simulink model "Drone2_simulink_old"  (R2024b)
settings: Solver=ode1be  StartTime=0.0  StopTime=1200  FixedStep=0.001  MaxStep=0.001  MinStep=0.00095  RelTol=1e-3
undefined symbols (not defined in the file): DiscIntNeverNeededParam, Environment, Newton, Raphson, Sim3dSensor, Vehicle, X, Y, Z
libraries: sm_lib x2953, nesl_utility x76, slpidlib x25, simulink x4, eeGeneralControl x4, matrix_library x3, rllib x2, sim3dlib x2, uavsim3dlib x2, dspstat3 x1, SignalEditorBlockLib x1, sharedutil x1
(part 21 of 21)

== matlab function Drone2_simulink_old/Controller (STA-Based)/New Control scheme with STA ==
  settings: updateMethod=DISCRETE  sampleTime=0.001
  data: state input; uc output; desired input; dt parameter; initialz input; tt input; b_out output; e output; ud_new output; parameter parameter; zd output; Env parameter; physical parameter; ld output; vd output; vd_dot output; eta1 output; e_dot output; term output; vzout output; S output; uc1 output; uc2 output; Aout output; AAout output
function [uc,b_out,e,ud_new,zd,ld,vd,vd_dot,eta1,e_dot,term,vzout,S,uc1,uc2,Aout,AAout] = Adaptive_Robust_Controller(state,desired, dt, initialz, tt,parameter,Env, physical)
%%%% defination
% x = states [z,p,u,w,q,lf,lr,lf_dot,lr_dot]
%  m = fixed mass
% m1 = moving mass 
% IB = Inertia tensor of 3*3
% rho = water density
% g = gravity (value in m/s^2)
% AS = syringe area
% ZS = CG location of z axis in each syringe [z1 z2 z3]
% l = length of vehicle/drone
% V = volume of drone
% rb = location of center of buoyancy from body frame [rbx rby rbz];
% RG = inital location of CG from body frame[ rgx rgy rgz];
% desired = target depth and pitch angle and velocities [z z_dot pitch
% pitch_rate]
% MATfile = file of disturnace jonswap.mat
% Parameters:    1x1 structure
%             
% 
% 
% fixed mass
% warning('on','MATLAB:singularMatrix');
% warning('on','MATLAB:nearlySingularMatrix');
% warning('on','MATLAB:illConditionedMatrix');
% dbstop if warning MATLAB:singularMatrix
% dbstop if warning MATLAB:nearlySingularMatrix
% dbstop if warning MATLAB:illConditionedMatrix


persistent isavail b vz vf_trim vb_trim AA A zr_prev


if isempty(isavail)
    b = zeros(2,1);%[0;0];
    A = zeros(2,1);%[0;0];
    AA = zeros(2,1);%[0;0];

    vz = zeros(2,1);%[0;0];
    vf_trim = 0;
    vb_trim = 0;
    zr_prev = desired(1);

    isavail = true;
end





m = physical.m;
IB = physical.IB;
Rsyringe = physical.Rsyringe;
RG = physical.RG;
rb = physical.rb;
l = physical.l;
ZS = physical.ZS;
Sden = physical.Sden;
maxb = physical.maxb;
minb = physical.minb;
rho = Env.rho;
g = abs(Env.g);
MaxBuoyancyVol = physical.MaxBuoyancyVol;
TT = physical.TimeConstant;


Srho = Sden*rho;





%% control gain constants

%<------- Backstepping with disturbance compensator error constant -------->

K1 = parameter.Backcomp.K1;
K2 = parameter.Backcomp.K2;
K22 = parameter.Backcomp.K22;
K2Z = parameter.Backcomp.K2Z;
K1SF = parameter.Backcomp.K1SF;
K2SF = parameter.Backcomp.K2SF;
K3SF =parameter.Backcomp.K3SF;
lb = parameter.Backcomp.lb;
alpha0 = parameter.Backcomp.alpha;
alpha1 = parameter.Backcomp.alpha1;
satphi = parameter.Backcomp.phisat;
satphi1 = parameter.Backcomp.phisat1;
K_trim = parameter.Backcomp.K_Trim;
K_rate = parameter.Backcomp.K_Rate;
EZDB = parameter.Backcomp.EZDB;
KP_trim = parameter.Backcomp.KP_Trim;
KP_rate = parameter.Backcomp.KP_Rate;
ETDB = parameter.Backcomp.ETDB;

%% extra
AS = pi*Rsyringe^2;
arc = [3 5];%[1 3 5];
jr = [3 5];
%% state Identification
% [m11,n1] = size(Dtrue);
% [m22,n22] = size(Ttrue);

Z = state(1);
r=0;y =0;
p = state(2);

u = state(3);
w = state(4);
q = state(5);
vel = [0;0;w];
omega = [0;q;0];



lf = state(6);
lr = state(7);

lf_dot = state(8);
lr_dot = state(9);



vel1 = [w;q];


%% Mass Matrix and coriollis matrix
Mdead = [m*eye(3) -m*skmatrix(RG); m*skmatrix(RG) IB ];  %% dead weight mass mo
Mdead11 = m*eye(3); Mdead12 = -m*skmatrix(RG); Mdead21=-Mdead12; Mdead22 = IB;
Cdead = [zeros(3)  -skmatrix(Mdead11*vel+Mdead12*omega);-skmatrix(Mdead11*vel+Mdead12*omega) -skmatrix(Mdead21*vel+Mdead22*omega)];

[MF1, MF1_dot ,CF1] = M_Mdot_C_Matrix(Srho,Rsyringe,lf,lf_dot,[(l-lf)/2; 0 ; ZS(1)],[-lf_dot/2 ;0 ;0],pi,omega,vel);
[MF2, MF2_dot ,CF2] = M_Mdot_C_Matrix(Srho,Rsyringe,lf,lf_dot,[(l-lf)/2; 0 ; ZS(2)],[-lf_dot/2 ;0 ;0],pi,omega,vel);
[MR, MR_dot ,CR] = M_Mdot_C_Matrix(Srho,Rsyringe,lr,lr_dot,[-(l-lr)/2; 0 ; ZS(3)],[lr_dot/2 ;0 ;0],0,omega,vel);





M = Mdead ;%+ MF1 +MF2 +MR;
C = Cdead;% + CF1 +CF2+ CR;

M_dot = MF1_dot+MF2_dot+MR_dot;


invM =  Mdead\eye(6); %(M+0.001*eye(6))\eye(6);

M = M(arc,arc);
M_dot = M_dot(arc,arc);
invM = invM(arc,arc);
C = C(arc,arc);



%% Making Transformation matrix

Rbw = [cos(p)*cos(y) sin(r)*sin(p)*cos(y)-cos(r)*sin(y)  cos(r)*sin(p)*cos(y)+sin(r)*sin(y);
    cos(p)*sin(y) sin(r)*sin(p)*sin(y)+cos(r)*cos(y)  cos(r)*sin(p)*sin(y)-sin(r)*cos(y);
    -sin(p) sin(r)*cos(p) cos(r)*cos(p)];

% Tbw = [1 sin(r)*tan(p) cos(r)*tan(p); 0 cos(r) -sin(r); 0 sin(r)/cos(p) cos(r)/cos(p)];

% J = [Rbw zeros(3); zeros(3) Tbw]; % 6*6 matrix

% J = J(jr,arc); %2*3 matrix [-sin(p) cos(p) 0; 0 0 1]
% invJ = pinv(J); % or simply j' as J*ji  = I2;      3*2 matrix 

% Jdot = [-cos(p)*q -sin(p)*q 0; 0 0 0];

%% Gravity Matrix
Fgn = [0;0;-Mdead(1,1)*g];
Fbn = [0;0;rho*MaxBuoyancyVol*g];

Fgb = Rbw'*Fgn;
Fbb = Rbw'*Fbn;
% G = -[Fgn+Fbn; cross(RG,Fgn)+cross(rb,Fbn)];
G = -[Fgb+Fbb; cross(RG,Fgb)+cross(rb,Fbb)]; % 6*1 matrix
G = G(arc); % 3*1 vector



%% desired 
if tt<=600
    z = desired(1);
else
    z = -2.5;
end

pd = desired(2);
tau = 4;

%% forward euler case
% zr_dot = (z-zr_prev)/tau;
% zd = zr_prev + dt*zr_dot;
% zr_prev = zd;

%% backward euler case
zd = (zr_prev+(z*dt/tau))/(1+(dt/tau));
zr_dot = (z-zd)/tau;
zr_prev = zd;

%% other desired velocities
eta_dot_d = [zr_dot;desired(4)];
% eta_dot_d = [desired(3);desired(4)];
eta_ddot_d = [desired(5);desired(6)];



        %% Backsteping Algorithm with distubance compensator gain
        e = [Z;p]-[zd;pd];
        
        %% first virtual controller \vd
                
        vd = eta_dot_d -K1*e;

        eta1 = vel1 - vd;
        
        
        e_dot = eta1-K1*e;
        
        vd_dot = eta_ddot_d-K1*e_dot;
        
        
        
        %% second virtual controller u

        % ud_new = (C*vel1+G + Damping - je-K2*eta1+M*vd_dot);
        term = abs(eta1).^0.5.*satfun(eta1,satphi1);



        ud_new = (C*vel1+G-M*(vd_dot-K2*eta1-K22*term+vz));
        % ud_new(1) = clipfunc(ud_new(1),10,0);
        % ud_new(2) = clipfunc(ud_new(2),1.5,-1.5);
        ud_new = reshape(ud_new,2,1);

        vzdot = -K2Z*satfun(eta1,satphi1);

        % vzdot = reshape(vzdot,2,1);
        vz = vz+vzdot*dt;
        vzout = vz;

%% New rule for finding lf and lr
        % K_Trim = 0.002; K_rate = 0.05;
        % EZDB = 0.05;
        % KP_trim = 0.0002; Kp_rate = 0.05;
        % ETDB = 0.05;

        dsum = ud_new(1)/(rho*AS*g);
        vf_fast = 0.25*dsum;
        vb_fast = 0.5*dsum;

        msum = ud_new(2)/(rho*AS*g);
        vf_pitch_fast = 0.25*msum;
        vb_pitch_fast = -0.15*msum; % change 0.5

        adapt_gate = 1/(1+K_rate*abs(eta1(1)));
        if abs(e(1))<EZDB
            adapt_gate = 0.25*adapt_gate;
        end
        dsum_trim = K_trim*e(1)*adapt_gate;

        pitch_gate = 1/(1+KP_rate*abs(eta1(2)));

        if abs(e(2))<ETDB
            pitch_gate = 0.2*pitch_gate;
        end
        msum_trim = KP_trim*e(2)*pitch_gate;

        msum_trim = clipfunc(msum_trim,0.01,-0.01);

        vf_trim_update = (0.25*dsum_trim-0.25*msum_trim)*dt;
        vb_trim_update = (0.25*dsum_trim+0.5*msum_trim)*dt;

        vf_trim = vf_trim+vf_trim_update;
        vb_trim = vb_trim+vb_trim_update;

        vf_cmd = vf_trim+vf_pitch_fast+vf_fast;
        vb_cmd = vb_fast+vb_trim+vb_pitch_fast;

        vf_cmd = clipfunc(vf_cmd,0.1,0.005);
        vb_cmd = clipfunc(vb_cmd,0.1,0.005);

        ld = [vf_cmd;vb_cmd];


% beta0 = [lf;lr];
        % newparams.rho = rho;
        % newparams.g = g;
        % newparams.AS = AS;
        % newparams.theta= p;
        % newparams.l = l;
        % newparams.ZS = ZS;

            % ld= solvebeta(AS,Srho,g,l,MF1,MF2,MR,ZS,p,ud_new,beta0,parameter.opts);
            % ld(1) = clipfunc(ld(1),0.1,0.005);
            % ld(2) = clipfunc(ld(2),0.1,0.005);
        %     ld = solve_beta_priority(ud_new,beta0,newparams,e(1));
            % ld = clip(ld,0.008,0.1);
 %% last actual control starts
            bb_dot = -lb*(b-ld);
            l_vec = [lf;lr];
            bbx = bb_dot*dt;
            b = b+bbx;
            b= reshape(b,2,1);
            assert(all(size(b) == [2,1]), 'b must be 2x1');
            b(1) = min(b(1), maxb);
            b(2) = min(b(2), maxb);
            b_out = b;
            eta2 = l_vec-b;
            eta2 =reshape(eta2,2,1);
assert(all(size(M)==[2 2]));
assert(all(size(eta1)==[2 1]));
assert(all(size(vd_dot)==[2 1]));
assert(all(size(vz)==[2 1]));


            %% actual control
            S = eta2+AA;
            S = reshape(S,2,1);

            uc1 = l_vec+TT*(bb_dot-K1SF*sig(eta2,alpha1));
            uc2 = -TT*(K2SF*abs(S).^0.5.*satfun(S,satphi)-A);
            uc = uc1+uc2;


            AA_update = K1SF*sig(eta2,alpha1);
            AA = AA+AA_update*dt;
            AAout = AA;

            A_update = -K3SF*satfun(S,satphi);
            A = A+ A_update*dt;
            Aout= A;
            assert(all(size(AA_update) == [2,1]), 'AA_update must be 2x1');

        

end



function [A] = skmatrix(r)

assert(isnumeric(r),'r must be numeric');
assert(isvector(r),'r must be a vector');
assert(numel(r)==3,'length of r must be 3')


A = [0    -r(3)   r(2);
     r(3)   0    -r(1);
    -r(2)  r(1)    0];
end


function [M , M_dot, C] = M_Mdot_C_Matrix(rho, radius, length,l_dot, r_vec,r_dot, theta,omega,vlin)
% Calculate the 6x6 added mass matrix of a cylinder (general case)
%
% Inputs:
%   rho          - Fluid density
%   radius       - Cylinder radius [m]
%   length       - Cylinder length [m] 
%   l_dot        - rate of change of cylinder length
%   r_vec        - 3x1 vector from reference point (body COM) to cylinder COM [m]
%   r_dot        - 3x1 vector d(r_vec)/dt
%   Theta        - Angle of z axis roatation to make axis aline in radian (cylinder local -> body frame)
%   omega        - 3x1 vector of angular velocity  in body frame
%   vlin         - 3x1 vector of linear velocity in body frame 
% Output:
%   M      - 6x6 mass matrix in body frame 
%   M_dot  - 6x6 m_dot matrix in body frame 
%  C       - 6x6 coriolis matrix in body frame 



%% checks


assert(size(r_dot,2)==1 && size(r_dot,1)==3,'r_dot must a 3x1 numreic column vector');
assert(size(r_vec,2)==1 && size(r_vec,1)==3,'r_dot must a 3x1 numreic column vector');
assert(size(omega,2)==1 && size(omega,1)==3,'r_dot must a 3x1 numreic column vector');
assert(size(vlin,2)==1 && size(vlin,1)==3,'r_dot must a 3x1 numreic column vector');



% Volume of cylinder
V = pi * radius^2 * length;

% theta = deg2rad(theta);  R maps the vectors expressed in CO frame into
% CG, i.e CG frame is obtained by rotating CO frame. -----> Vcg = R*Vco
% frame.
R = [cos(theta) -sin(theta) 0;
    sin(theta) cos(theta) 0;
    0 0 1];

% Displaced fluid mass
m_disp = rho * V;

% Linear added mass matrix (local frame)
% Axial direction: x-axis of cylinder
% Transverse directions: y,z axes
M11_local = eye(3) * m_disp;

% Added inertia of fluid about cylinder COM in local frame
% Use standard moments of inertia formulas for a solid cylinder filled with fluid mass (added mass)
% Here, assuming fluid added mass distributed as cylinder mass with coefficients
% For fluid added inertia, multiply by coefficients as well

% Moments of inertia of solid cylinder about its center along principal axes
I_xx = 0.5 * m_disp * radius^2;                   % about cylinder axis (axial)
I_yy = (1/12) * m_disp * (3*radius^2 + length^2); % about transverse axis y
I_zz = I_yy;                                      % about transverse axis z

% Multiply moments by added mass coefficients
I_g_local = diag([I_xx, I_yy, I_zz]);

% Construct cross product matrix of r_vec
S_r = skmatrix(r_vec);

% Cross coupling matrices
% M12 = -m_disp * S_r;
% M21 = -M12;

% Rotate inertia to body frame
I_new = R' * I_g_local * R;

% Apply parallel axis theorem to inertia matrix about reference point
I_b = I_new + m_disp * (S_r * S_r');

% Rotate linear added mass matrix to body frame as well
M11 = R' * M11_local * R;
M12 = M11*S_r;
M21 = -M12;

% Assemble full 6x6 added mass matrix
M = [M11, M12;
     M21, I_b];



%% calculation of M dot

m1dot = rho*pi * radius^2 *l_dot;
M11dot_local = m1dot*eye(3);
M11dot = R*M11dot_local*R';
M12dot = -m1dot*skmatrix(r_vec)-m_disp*skmatrix(r_dot);
M21dot = -M12;

Ixx_dot = 0.5*rho*pi*radius^2*l_dot;
Iyy_dot = 1/12*(m1dot*(3*(r_vec'*r_vec)+length*length)+m_disp*(2*l_dot));
Izz_dot = Iyy_dot;

Idot_global = diag([Ixx_dot, Iyy_dot, Izz_dot]);


Idot = R*Idot_global*R'; 

M22dot = Idot + m1dot*(r_vec'*r_vec*eye(3)-r_vec*r_vec')+m_disp*(2*r_vec'*r_dot*eye(3) - (r_dot*r_vec'+r_vec*r_dot'));



M_dot = [M11dot M12dot; M21dot M22dot];


%% calcu lation of C


S_om = skmatrix(omega);
S_v = skmatrix(vlin);

adT = [S_om -S_v; zeros(3) S_om];

% C = -adT'*M+ M_dot;  %initally adT*M+M_dot


%% second way
% C = hdot'*M*h+h'*M*hdot+h'*Mdot*H+CC(v)*H'MH

Mnew = [M11_local zeros(3); zeros(3) ,I_g_local];
H = [R -R*skmatrix(r_vec);zeros(3) R*eye(3)];
Hdot = [zeros(3) -R*skmatrix(r_dot); zeros(3) zeros(3)];
M11CGdot = m1dot*eye(3);
M22Cgdot = diag([Ixx_dot, Iyy_dot, Izz_dot]);
Mdot = [M11CGdot zeros(3);zeros(3) M22Cgdot];
CCv = [skmatrix(omega) zeros(3); skmatrix(vlin) skmatrix(omega)];
C = Hdot'*Mnew*H +H'*Mdot*H +H'*M*Hdot +CCv*H'*M*H;

end


function beta = solvebeta(AS,rho,g,l,MF1,MF2,MR,ZS,theta, v, beta0, opts)
%SOLVE_BETA  Solve h(x, beta) = v for beta using Newton + LM + fallback
%
%   Inputs:
%       h_fun  : function handle, h_fun(x, beta) returns 2x1 vector
%       Jh_fun : function handle, Jh_fun(x, beta) returns 2x2 Jacobian wrt beta
%       x      : system state
%       v      : desired virtual input
%       beta0  : warm-start initial guess (2x1)
%       opts   : options struct with fields:
%                   .maxIter     (default 10)
%                   .tol_r       (default 1e-6)
%                   .tol_beta    (default 1e-6)
%                   .lambdaLM0   (default 1e-6)
%                   .regPI       (default 1e-6)
%                   .beta_min    (optional box constraint)
%                   .beta_max
%
%   Outputs:
%       beta   : solved beta
%       info   : struct with fields:
%                   .iterations
%                   .residual
%                   .converged
%                   .usedFallback
%
%   Jay's UAV–AUV Hybrid Control Project (PHD_DRONE)
%   ----------------------------------------------------

% h_fun = [(MF1(1,1)+MF2(1,1)+MR(1,1))*g*sin(theta);  -(MF1(1,1)+MF2(1,1)+MR(1,1))*g*cos(theta); (MF1(1,1)+MF2(1,1))*g*(cos(theta)*((l-beta_trial(1))/2)+ZS(1)*sin(theta))+(MR(1,1))*g*(cos(theta)*(-(l-beta_trial(2))/2)+ZS(3)*sin(theta))];

% Jh_func = [rho*g*AS*2*sin(theta) rho*g*AS*sin(theta); -rho*g*2*cos(theta) -rho*g*AS*cos(theta); rho*g*AS*((l-2*beta(1))*cos(zz)+2*ZS(1)*sin(theta))  rho*g*AS*(0.5*(l-2*beta(2))*cos(theta)+ZS(3)*sin(theta)) ];


%% Default options
if ~isfield(opts,'MaxIter');    opts.MaxIter  = 10;     end
if ~isfield(opts,'tol_r');      opts.tol_r    = 1e-6;   end
if ~isfield(opts,'tol_beta');   opts.tol_beta = 1e-6;   end
if ~isfield(opts,'lambdaLM0');  opts.lambdaLM0 = 1e-6;  end
if ~isfield(opts,'regPI');      opts.regPI    = 1e-6;   end

beta = beta0;
lambda = opts.lambdaLM0;
% usedFallback = false;

%% Iterative solve
for k = 1:opts.MaxIter
    
    % r = [(MF1(1,1)+MF2(1,1)+MR(1,1))*g*sin(theta);  -(MF1(1,1)+MF2(1,1)+MR(1,1))*g*cos(theta); (MF1(1,1)+MF2(1,1))*g*(cos(theta)*((l-beta(1))/2)+ZS(1)*sin(theta))+(MR(1,1))*g*(cos(theta)*(-(l-beta(2))/2)+ZS(3)*sin(theta))] - v;           % residual
     r = [  -(MF1(1,1)+MF2(1,1)+MR(1,1))*g*cos(theta); (MF1(1,1)+MF2(1,1))*g*(cos(theta)*((l-beta(1))/2))+(MR(1,1))*g*(cos(theta)*(-(l-beta(2))/2))] - v;           % residual
    
    % if norm(r) < opts.tol_r
    %     break;
    % end
    
    % Jacobian 2x3
    % J = [rho*g*AS*2*sin(theta) rho*g*AS*sin(theta); -rho*g*2*AS*cos(theta) -rho*g*AS*cos(theta); rho*g*AS*((l-2*beta(1))*cos(theta)+2*ZS(1)*sin(theta))  rho*g*AS*(-0.5*(l-2*beta(2))*cos(theta)+ZS(3)*sin(theta)) ];
    J = [-rho*g*2*AS -rho*g*AS; rho*g*AS*((l-2*beta(1))*cos(theta))  rho*g*AS*(-0.5*(l-2*beta(2))*cos(theta)) ];
    % LM step: (J'J + lambda I) delta = -J' r
    % lambda = max(lambda, 1e-6);   % keeps it from becoming too small

    A = J'*J + lambda * eye(2);
    % A = A+ 1e-8*eye(2); 
    gg = J' * r;
    
   if rcond(A) < 1e-12 || any(isnan(A(:))) || any(isinf(A(:)))
       delta = pinv(A) * gg;
   else
       delta = A \ gg;
   end
%% SVD decomposition method
    % [U, S, V] = svd(J, 'econ');
    % S_d = diag(S);
    % S_reg = S_d ./ (S_d.^2 + lambda);   % LM update in SVD domain
    % delta = -V * diag(S_reg) * U' * r;

    
    
    % delta = -A \ g;
    beta_trial = beta + delta;
    
    % Enforce optional bounds
    if isfield(opts,'beta_min')
        for i =1:2
            beta_trial(i) = max(beta_trial(i), opts.beta_min);
        end
    end
    if isfield(opts,'beta_max')
        for i =1:2
            beta_trial(i) = min(beta_trial(i), opts.beta_max);
        end
    end
    
    % Check residual improvement
    % r_trial = [(MF1(1,1)+MF2(1,1)+MR(1,1))*g*sin(theta);  -(MF1(1,1)+MF2(1,1)+MR(1,1))*g*cos(theta); (MF1(1,1)+MF2(1,1))*g*(cos(theta)*((l-beta_trial(1))/2)+ZS(1)*sin(theta))+(MR(1,1))*g*(cos(theta)*(-(l-beta_trial(2))/2)+ZS(3)*sin(theta))] - v;
     r_trial = [-(MF1(1,1)+MF2(1,1)+MR(1,1))*g; (MF1(1,1)+MF2(1,1))*g*(cos(theta)*((l-beta(1))/2))+(MR(1,1))*g*(cos(theta)*(-(l-beta(2))/2))] - v;           % residual
    if norm(r_trial) < norm(r)       % accept step
        beta = beta_trial;
        lambda = lambda / 10;
        
        if norm(delta) < opts.tol_beta
            break;
        end
        
    else                             % reject step
        lambda = lambda * 10;
        
        % If lambda becomes huge → fallback
        if lambda > 1e6
            % usedFallback = true;
            % Regularized pseudo-inverse step
            delta_pi = -(J'*J + opts.regPI*eye(2)) \ (J'*r);
            beta = beta + delta_pi;
            break;
        end
    end
end
end

function beta = solvebeta_pinv(AS,rho,g,l,MF1,MF2,MR,ZS,theta, v,beta0, opts)
%SOLVE_BETA  Solve h(x, beta) = v for beta using Newton + LM + fallback
%
%   Inputs:
%       h_fun  : function handle, h_fun(x, beta) returns 2x1 vector
%       Jh_fun : function handle, Jh_fun(x, beta) returns 2x2 Jacobian wrt beta
%       x      : system state
%       v      : desired virtual input
%       beta0  : warm-start initial guess (2x1)
%       opts   : options struct with fields:
%                   .maxIter     (default 10)
%                   .tol_r       (default 1e-6)
%                   .tol_beta    (default 1e-6)
%                   .lambdaLM0   (default 1e-6)
%                   .regPI       (default 1e-6)
%                   .beta_min    (optional box constraint)
%                   .beta_max
%
%   Outputs:
%       beta   : solved beta
%       info   : struct with fields:
%                   .iterations
%                   .residual
%                   .converged
%                   .usedFallback
%
%   Jay's UAV–AUV Hybrid Control Project (PHD_DRONE)
%   ----------------------------------------------------

% h_fun = [(MF1(1,1)+MF2(1,1)+MR(1,1))*g*sin(theta);  -(MF1(1,1)+MF2(1,1)+MR(1,1))*g*cos(theta); (MF1(1,1)+MF2(1,1))*g*(cos(theta)*((l-beta_trial(1))/2)+ZS(1)*sin(theta))+(MR(1,1))*g*(cos(theta)*(-(l-beta_trial(2))/2)+ZS(3)*sin(theta))];

% Jh_func = [rho*g*AS*2*sin(theta) rho*g*AS*sin(theta); -rho*g*2*cos(theta) -rho*g*AS*cos(theta); rho*g*AS*((l-2*beta(1))*cos(zz)+2*ZS(1)*sin(theta))  rho*g*AS*(0.5*(l-2*beta(2))*cos(theta)+ZS(3)*sin(theta)) ];


%% Default options
% if ~isfield(opts,'MaxIter');    opts.MaxIter  = 10;     end
% if ~isfield(opts,'tol_r');      opts.tol_r    = 1e-6;   end
% if ~isfield(opts,'tol_beta');   opts.tol_beta = 1e-6;   end
% if ~isfield(opts,'lambdaLM0');  opts.lambdaLM0 = 1e-6;  end
% if ~isfield(opts,'regPI');      opts.regPI    = 1e-6;   end

beta = beta0;
% lambda = opts.lambdaLM0;
lambda = 0;
%% Iterative solve
for k = 1:opts.MaxIter
    beta_prev = beta;
    % r = [(MF1(1,1)+MF2(1,1)+MR(1,1))*g*sin(theta);  -(MF1(1,1)+MF2(1,1)+MR(1,1))*g*cos(theta); (MF1(1,1)+MF2(1,1))*g*(cos(theta)*((l-beta(1))/2)+ZS(1)*sin(theta))+(MR(1,1))*g*(cos(theta)*(-(l-beta(2))/2)+ZS(3)*sin(theta))] - v;           % residual
    r = [  -(MF1(1,1)+MF2(1,1)+MR(1,1))*g*cos(theta); (MF1(1,1)+MF2(1,1))*g*(cos(theta)*((l-beta(1))/2))+(MR(1,1))*g*(cos(theta)*(-(l-beta(2))/2))] - v;           % residual
    
    % Jacobian 2x3
    % J = [rho*g*AS*2*sin(theta) rho*g*AS*sin(theta); -rho*g*2*AS*cos(theta) -rho*g*AS*cos(theta); rho*g*AS*((l-2*beta(1))*cos(theta)+2*ZS(1)*sin(theta))  rho*g*AS*(-0.5*(l-2*beta(2))*cos(theta)+ZS(3)*sin(theta)) ];
    J = [-rho*g*2*AS -rho*g*AS; rho*g*AS*((l-2*beta(1))*cos(theta))  rho*g*AS*(-0.5*(l-2*beta(2))*cos(theta)) ];
    beta = beta-(J.'*J+lambda*eye(2))\(J.'*r);
    

    r = [-(MF1(1,1)+MF2(1,1)+MR(1,1))*g; (MF1(1,1)+MF2(1,1))*g*(cos(theta)*((l-beta(1))/2))+(MR(1,1))*g*(cos(theta)*(-(l-beta(2))/2))] - v;           % residual

    if all(abs(beta-beta_prev) < 1e-3) && norm(r)<opts.tol_r
        break
    end


end
 % alpha = opts.alpha;   
 % beta = alpha*beta+(1-alpha)*beta0;   
    % Enforce optional bounds
    % if isfield(opts,'beta_min')
    %     for i=1:length(beta)
    %         beta(i) = min(opts.beta_max,max(beta(i), opts.beta_min));
    %     end
    % end
    % if isfield(opts,'beta_max')
    %     for i=1:length(beta)
    %         beta(i) = min(beta(i), opts.beta_max);
    %     end
    % end 
end


%% Prepare info
% info.iterations = k;
% info.residual = norm([(MF1(1,1)+MF2(1,1)+MR(1,1))*g*sin(theta);  -(MF1(1,1)+MF2(1,1)+MR(1,1))*g*cos(theta); (MF1(1,1)+MF2(1,1))*g*(cos(theta)*((l-beta(1))/2)+ZS(1)*sin(theta))+(MR(1,1))*g*(cos(theta)*(-(l-beta(2))/2)+ZS(3)*sin(theta))]-v);
% % info.converged = info.residual < opts.tol_r;
% info.usedFallback = usedFallback;



function y =clipfunc(x,Max,Min)
y = min(Max,max(x,Min));
end



function h = compute_force(beta, params)
% Computes force vector h(beta) = [Fx; Fz; M]

rho   = params.rho;
AS    = params.AS;
g     = params.g;
theta = params.theta;
l     = params.l;
ZS    = params.ZS;

% ----- Mass terms -----
MF = rho * AS * beta(1);   % front (2 syringes)
MR = rho * AS * beta(2);   % rear

% ----- Force magnitude -----
A = g * (2*MF + MR);

% ----- Force components -----
Fx = A * sin(theta);
Fz = -A * cos(theta);

% ----- Moment -----
M = (2*MF)*g*( cos(theta)*((l - beta(1))/2) + ZS(1)*sin(theta) ) ...
  + (MR)*g*( cos(theta)*(-(l - beta(2))/2) + ZS(3)*sin(theta) );

% ----- Output -----
h = [Fx; Fz; M];

end


function J = compute_J(beta, params)

rho   = params.rho;
AS    = params.AS;
g     = params.g;
theta = params.theta;
l     = params.l;
ZS    = params.ZS;

k = rho * AS;

b1 = beta(1);
b2 = beta(2);

J = zeros(3,2);

%% ===== Force part =====

dA_db1 = 2 * k * g;
dA_db2 = 1 * k * g;

J(1,1) = dA_db1 * sin(theta);
J(1,2) = dA_db2 * sin(theta);

J(2,1) = -dA_db1 * cos(theta);
J(2,2) = -dA_db2 * cos(theta);

%% ===== Moment part (CORRECT NONLINEAR) =====

J(3,1) = k*g*cos(theta)*(l - 2*b1) ...
       + 2*k*g*ZS(1)*sin(theta);

J(3,2) = -0.5*k*g*cos(theta)*(l - 2*b2) ...
       + k*g*ZS(3)*sin(theta);

end



function beta = solve_beta_priority(ud, beta_prev, params, e_z)

beta = beta_prev;

rho = params.rho;
AS  = params.AS;
g   = params.g;
theta = params.theta;

alpha = 0.005;
lambda = 3;

% ----- weights -----
k = 5;
wz = 1;
wx = exp(-k*abs(e_z));
wm = exp(-k*abs(e_z));

W = diag([wx, wz, wm]);

for i = 1:5

    h = compute_force(beta, params);
    e = h - ud;

    J = compute_J(beta, params);

    % 🔥 weighted gradient
    grad = J' * (W * e) + lambda*(beta - beta_prev);

    beta = beta - alpha * grad;

    % bounds
    beta(1) = min(max(beta(1),0.005),0.1);
    beta(2) = min(max(beta(2),0.005),0.1);

end

end

function y = satfun(x, phi)
%#codegen
% Element-wise saturation: y = sat(x/phi)

    % Small value to avoid division by zero
    eps_val = 1e-6;
     assert(all(phi(:) > 0), 'phi must be > 0');

    % Ensure phi is not zero (element-wise safe)
    phi_safe = phi + (phi == 0) * eps_val;

    % Element-wise division
    u = x ./ phi_safe;

    % Saturation
    y = min(max(u, -1), 1);
end


function y = sig(x, alpha)
%#codegen

% Validate alpha (codegen-safe)
if alpha <= 0 || alpha >= 1
    error('alpha must be in (0,1)');
end

% Preallocate
y = zeros(size(x));

% Element-wise operation
for i = 1:numel(x)
    if x(i) > 0
        y(i) = x(i)^alpha;
    elseif x(i) < 0
        y(i) = -((-x(i))^alpha);
    else
        y(i) = 0;
    end
end
end
% function [uc,b_out,e,ud_new,zd] = Adaptive_Robust_Controller(state,desired, k1e1, k1e2, k2e1, k2e2, k2e3, k3e1, k3e2, d1, d2, g1, g2, g3, sigma, m, IB, Rsyringe, RG, rb, l, ZS, lb,MaxIter, lambdaLM0,tol_r, tol_beta, minb, maxb,Sden, rho, dt, g, MaxBuoyancyVol,sigma1, alpha, initialz, tt,Ctrlchoice)

== matlab function Drone2_simulink_old/Hydrostatic & Hydrodynamic Effects/Buoyancy Force/MATLAB Function ==
  data: Z input; Factor output; a input; b input; y_a input; y_b input; reverse input
function Factor = quadratic_map(Z, a, b, y_a, y_b, reverse)
    % Quadratic mapping from [a, b] to [y_a, y_b]
    % reverse = 0 -> Normal mapping (a -> y_a, b -> y_b)
    % reverse = 1 -> Reverse mapping (a -> y_b, b -> y_a)
    
    c = (y_b - y_a) / (b - a)^2;
    
    if reverse
        Factor = y_b - c * (Z - a).^2;
    else
        Factor = c * (Z - a).^2 + y_a;
    end
end

== matlab function Drone2_simulink_old/Hydrostatic & Hydrodynamic Effects/Wind force/wind_disturbance ==
  settings: updateMethod=DISCRETE
  data: t input; vx output; v_mean input; v_max input; vy output; vz output
function [vx, vy, vz] = windVelocity(t,v_mean,v_max)
% Deterministic wind with stochastic component
 % mean wind in x
v_turb = 0.5 * sin(0.1 * t) .* randn(3,1);  % small gusts
v_wind = v_mean + v_turb;

% Optionally clamp:
if norm(v_wind) > v_max
    v_wind = 3 * v_wind / norm(v_wind);
end
vx = v_wind(1);
vy = v_wind(2);
vz = v_wind(3);
end
